simulink model "prova_simu_clock"  (Simulink 7.7)
settings: Solver=FixedStepDiscrete  SolverMode=SingleTasking  StartTime=0.0  StopTime=Tf  FixedStep=Ts  RelTol=1e-3
values from neighbouring files (symbols this model uses):
  Ts = 0.1    [receiver_clock_error.m]
undefined symbols (not defined in the file or in its folder): afz, az, bfz, bz, cfz, cz, dfz, DiscIntNeverNeededParam, dz
libraries: simulink x1
settings Model: Creator=tiziana.ingrassia  LastModifiedBy=tiziana.ingrassia
settings DataIOCC: LimitDataPoints=off

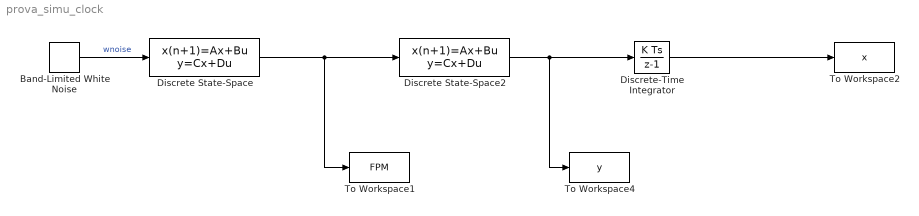
== system prova_simu_clock ==
  Band-Limited White Noise : simulink/Sources/Band-Limited White Noise  SystemSampleTime=-1  Cov=1/2  Ts=Ts  seed=[546716598]
  Discrete State-Space : DiscreteStateSpace  A=az  B=bz  C=cz  D=dz  SampleTime=-1
  Discrete State-Space2 : DiscreteStateSpace  A=afz  B=bfz  C=cfz  D=dfz  SampleTime=-1
  Discrete-Time Integrator : DiscreteIntegrator  SampleTime=-1  ICPrevOutput=DiscIntNeverNeededParam  ICPrevScaledInput=DiscIntNeverNeededParam
  To Workspace1 : ToWorkspace  VariableName=FPM  SampleTime=-1  SaveFormat=Array
  To Workspace2 : ToWorkspace  VariableName=x  SampleTime=-1  SaveFormat=Array
  To Workspace4 : ToWorkspace  VariableName=y  SampleTime=-1  SaveFormat=Array
  wires:
  Discrete-Time Integrator/1 -> To Workspace2/1
  Discrete State-Space2/1 -> Discrete-Time Integrator/1, To Workspace4/1
  Discrete State-Space/1 -> To Workspace1/1, Discrete State-Space2/1
  Band-Limited White Noise/1 -> Discrete State-Space/1  "wnoise"
